simulink model "assignment1_b"  (R2024b)
settings: Solver=VariableStepAuto  StartTime=0.0  StopTime=inf  RelTol=1e-3
settings Model: Creator=ANURRADHA  LastModifiedBy=ANURRADHA

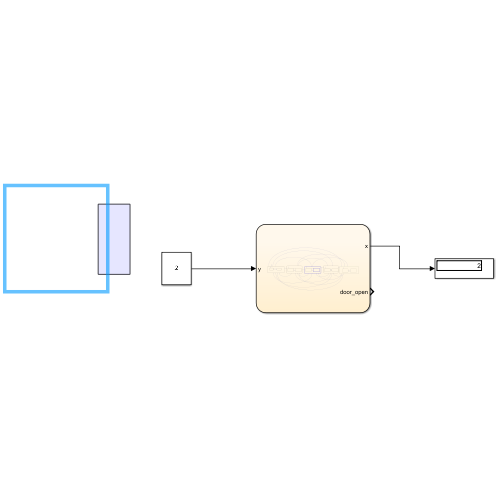
[thumbnail: Simulink's stored preview of the top-level diagram]
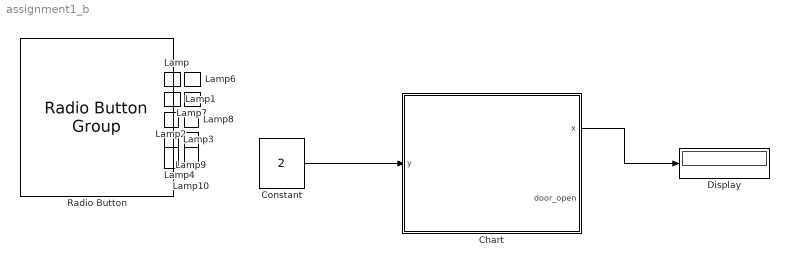
== system assignment1_b ==
  Chart : Stateflow chart  TreatAsAtomicUnit=on
  Constant : Constant  Value=2
  Display : Display
  Lamp{,1..4,6..10} (10 alike) : LampBlock  LabelPosition=Hide
  Radio Button : RadioButtonGroup  LabelPosition=Hide  SelectedLabel=SECOND_FLOOR  ButtonGroupName=ELEVATOR
      settings: Values={{'GROUND_FLOOR', 'FIRST_FLOOR', 'SECOND_FLOOR', 'THIRD_FLOOR', 'FOURTH_FLOOR'}, [0 1 2 3 4]}
  wires:
  Constant/1 -> Chart/1(y)
  Chart/1(x) -> Display/1

== stateflow chart assignment1_b/Chart ==
  state F_3
    x=3;
    state closed_1
      door_open =0;
    state open_1
      door_open =1;
    (default) -> F_3.closed_1
    F_3.open_1 -> F_3.closed_1 : [x~=3]{after(10,sec)}
    F_3.closed_1 -> F_3.open_1 : [x==3]{after(10,sec)}
  state F_1
    x=1;
    state closed_1
      door_open =0;
    state open_1
      door_open =1;
    (default) -> F_1.closed_1
    F_1.open_1 -> F_1.closed_1 : [x~=1]{after(10,sec)}
    F_1.closed_1 -> F_1.open_1 : [x==1]{after(10,sec)}
  state F_0
    x=0;
    state closed_1
      door_open =0;
    state open_1
      door_open =1;
    (default) -> F_0.closed_1
    F_0.open_1 -> F_0.closed_1 : [x~=0]{after(10,sec)}
    F_0.closed_1 -> F_0.open_1 : [x==0]{after(10,sec)}
  state F_4
    x=4;
    state closed_1
      door_open =0;
    state open_1
      door_open =1;
    (default) -> F_4.closed_1
    F_4.open_1 -> F_4.closed_1 : [x~=4]{after(10,sec)}
    F_4.closed_1 -> F_4.open_1 : [x==4]{after(10,sec)}
  state F_2
    x=2;
    state closed_1
      door_open =0;
    state open_1
      door_open =1;
    (default) -> F_2.closed_1
    F_2.open_1 -> F_2.closed_1 : [x~=2]{after(10,sec)}
    F_2.closed_1 -> F_2.open_1 : [x==2]{after(10,sec)}
  F_0 -> F_4 [order 4] : [y==4]{after(80,sec)}
  F_0 -> F_3 [order 2] : [y==3]{after(60,sec)}
  F_1 -> F_4 [order 4] : [y==4]{after(60,sec)}
  F_0 -> F_2 [order 3] : [y==2]{after(40,sec)}
  F_2 -> F_4 [order 1] : [y==4]{after(40,sec)}
  F_1 -> F_3 [order 3] : [y==3]{after(40,sec)}
  (default) -> F_0
  F_3 -> F_4 [order 1] : [y==4]{after(20,sec)}
  F_2 -> F_3 [order 2] : [y==3]{after(20,sec)}
  F_0 -> F_1 [order 1] : [y==1]{after(40,sec)}
  F_1 -> F_2 [order 1] : [y==2]{after(20,sec)}
  F_2 -> F_0 [order 4] : [y==0]{after(40,sec)}
  F_3 -> F_0 [order 4] : [y==0]{after(60,sec)}
  F_4 -> F_0 [order 1] : [y==0]{after(80,sec)}
  F_1 -> F_0 [order 2] : [y==0]{after(20,sec)}
  F_3 -> F_1 [order 3] : [y==1]{after(40,sec)}
  F_3 -> F_2 [order 2] : [y==2]{after(20,sec)}
  F_4 -> F_3 [order 4] : [y==3]{after(20,sec)}
  F_2 -> F_1 [order 3] : [y==1]{after(20,sec)}
  F_4 -> F_1 [order 2] : [y==1]{after(60,sec)}
  F_4 -> F_2 [order 3] : [y==2]{after(40,sec)}
  data: x output; y input; door_open output double
